simulink model "RemoteMicrogrid"  (R2025a)
settings: Solver=FixedStepAuto  StartTime=0.0  StopTime=8  FixedStep=Ts  MaxStep=1e-3  RelTol=1e-3
PreLoadFcn:
  | RemoteMicrogridInputData
undefined symbols (not defined in the file): BESS, ControlRoom, DiscIntNeverNeededParam, Grid, Load, Machine, Microgrid, MicrogridStatus, PV, relay1, T_on, Ts
libraries: ee_lib x53, fl_lib x39, eeGeneralControl x30, simulink x30, nesl_utility x26, nesl_utility_internal x19, slpidlib x7, eeTransforms x5, eeRmsMeasurement x4, eeTotalHarmonicDistorsion x4, batteryecm_lib x2, simulink_extras x2
(part 5 of 6)

== system RemoteMicrogrid/Diesel Substation, BESS, & Microgrid Controller/Microgrid Controller/Microgrid Supervisory Control/Transition and Dispatch Control/On.Unplanned_Islanding ==
  " Demux " : Demux  Outputs=1
  " Ground " : Ground
  " SFunction " : S-Function  Tag=Stateflow S-Function 9  FunctionName=sf_sfun  PortCounts=[1 6]  SFunctionDeploymentMode=off  EnableBusSupport=off
  " Terminator " : Terminator
  PCC : Outport
  loadDispatch : Outport  Port=2
  loadF2A : Outport  Port=3
  loadF2B : Outport  Port=4
  emergencyDispatch : Outport  Port=5
  wires:
  " SFunction "/2 -> PCC/1  "PCC"
  " SFunction "/3 -> loadDispatch/1  "loadDispatch"
  " SFunction "/4 -> loadF2A/1  "loadF2A"
  " SFunction "/5 -> loadF2B/1  "loadF2B"
  " SFunction "/6 -> emergencyDispatch/1  "emergencyDispatch"
  " Ground "/1 -> " SFunction "/1
  " Demux "/1 -> " Terminator "/1
  " SFunction "/1 -> " Demux "/1

== system RemoteMicrogrid/Operator Control Room/Microgrid Control/Protection & Power Tracking/Overcurrent relay ==
  Inport : Inport
  Data Type Conversion : DataTypeConversion  OutDataTypeStr=double  SaturateOnIntegerOverflow=off  RndMeth=Floor
  Delay : Delay  DelayLength=1
  Earth Protection Unit : Subsystem
  Enable : Gain  Gain=protectionEnable
  Fourier Analysis : Subsystem
  Mux1 : Mux  Inputs=2
  OR1 : Logic  Operator=OR  IconShape=distinctive  AllPortsSameDT=off  OutDataTypeStr=boolean
  Phase Protection Unit : Subsystem
  Trip Signal : Outport
  Relay Status : Outport  Port=2
  wires:
  Data Type Conversion/1 -> Enable/1
  Enable/1 -> Delay/1
  Delay/1 -> Trip Signal/1
  [Rer] -> Mux1/2
  [Rph] -> Mux1/1
  Mux1/1 -> Relay Status/1
  OR1/1 -> Data Type Conversion/1
  Inport/1 -> Fourier Analysis/1(Current)
  Fourier Analysis/1(Magnitude) -> [mag]
  Fourier Analysis/2(Angle) -> [iphi]
  [mag] -> Phase Protection Unit/1(Current)
  [mag] -> Earth Protection Unit/1(Mag)
  [iphi] -> Earth Protection Unit/2(Phi)
  Phase Protection Unit/1(Trip Signal) -> OR1/1, [Rph]
  Earth Protection Unit/1(Trip Signal) -> [Rer], OR1/2

== system RemoteMicrogrid/Operator Control Room/Performance and Power Quality/Load Performance /Subsystem4 ==
  Voltage : Inport
  Change Detector : eeGeneralControl/Change Detector  VariantControl=Variant1  LabelModeActiveChoice=Discrete  ChangeType=Rising edge  x0=0  Ts=Ts
  Change Detector1 : eeGeneralControl/Change Detector  VariantControl=Variant1  LabelModeActiveChoice=Discrete  ChangeType=Rising edge  x0=0  Ts=Ts
  Compare To Constant2 : simulink/Logic and Bit Operations/Compare To Constant  relop=<=  const=Microgrid.LoadVolatgeRMSLow  OutDataTypeStr=boolean
  Compare To Constant3 : simulink/Logic and Bit Operations/Compare To Constant  relop=>  const=Microgrid.LoadVolatgeRMSHigh  OutDataTypeStr=boolean
  VoltageLow : Outport
  VoltageHigh : Outport  Port=2
  wires:
  Change Detector/1 -> VoltageLow/1
  Compare To Constant2/1 -> Change Detector/1
  Voltage/1 -> Compare To Constant3/1, Compare To Constant2/1
  Change Detector1/1 -> VoltageHigh/1
  Compare To Constant3/1 -> Change Detector1/1

== system RemoteMicrogrid/Operator Control Room/Performance and Power Quality/Load Performance /start at 0.2 s2 ==
  In1 : Inport
  Constant : Constant
  Step : Step  Time=2.5  SampleTime=Ts
  Switch : Switch  Criteria=u2 > Threshold  Threshold=0.5  SaturateOnIntegerOverflow=off  InputSameDT=off
  u : Outport
  wires:
  In1/1 -> Switch/1
  Switch/1 -> u/1
  Constant/1 -> Switch/3
  Step/1 -> Switch/2

== system RemoteMicrogrid/Operator Control Room/Performance and Power Quality/Load Performance /start at 0.2 s4 ==
  In1 : Inport
  Constant : Constant  Value=0.491
  Step : Step  Time=2.5  SampleTime=Ts
  Switch : Switch  Criteria=u2 > Threshold  Threshold=0.5  SaturateOnIntegerOverflow=off  InputSameDT=off
  u : Outport
  wires:
  In1/1 -> Switch/1
  Switch/1 -> u/1
  Constant/1 -> Switch/3
  Step/1 -> Switch/2

== system RemoteMicrogrid/Operator Control Room/Performance and Power Quality/Load Performance /start at 0.2 s5 ==
  In1 : Inport
  Constant : Constant  Value=75
  Step : Step  Time=2.5  SampleTime=Ts
  Switch : Switch  Criteria=u2 > Threshold  Threshold=0.5  SaturateOnIntegerOverflow=off  InputSameDT=off
  u : Outport
  wires:
  Step/1 -> Switch/2
  Constant/1 -> Switch/3
  Switch/1 -> u/1
  In1/1 -> Switch/1

== system RemoteMicrogrid/Operator Control Room/Performance and Power Quality/Loss Calculation/start at 2.5 s ==
  ReactivePower : Inport
  Constant : Constant
  Step : Step  Time=2.5  SampleTime=Ts
  Switch : Switch  Criteria=u2 > Threshold  Threshold=0.5  SaturateOnIntegerOverflow=off  InputSameDT=off
  u : Outport
  wires:
  ReactivePower/1 -> Switch/1
  Switch/1 -> u/1
  Constant/1 -> Switch/3
  Step/1 -> Switch/2

== system RemoteMicrogrid/Operator Control Room/Performance and Power Quality/Loss Calculation/start at 2.5 s1 ==
  ActivePower : Inport
  Constant : Constant
  Step : Step  Time=2.5  SampleTime=Ts
  Switch : Switch  Criteria=u2 > Threshold  Threshold=0.5  SaturateOnIntegerOverflow=off  InputSameDT=off
  u : Outport
  wires:
  Step/1 -> Switch/2
  Constant/1 -> Switch/3
  Switch/1 -> u/1
  ActivePower/1 -> Switch/1

== system RemoteMicrogrid/Operator Control Room/Performance and Power Quality/Microgrid Power Quality /Subsystem ==
  Frequency : Inport
  Change Detector : eeGeneralControl/Change Detector  VariantControl=Variant1  LabelModeActiveChoice=Discrete  ChangeType=Rising edge  x0=0  Ts=Ts
  Change Detector1 : eeGeneralControl/Change Detector  VariantControl=Variant1  LabelModeActiveChoice=Discrete  ChangeType=Rising edge  x0=0  Ts=Ts
  Compare To Constant2 : simulink/Logic and Bit Operations/Compare To Constant  relop=<  const=Microgrid.FrequencyLow  OutDataTypeStr=boolean
  Compare To Constant3 : simulink/Logic and Bit Operations/Compare To Constant  relop=>  const=Microgrid.FrequencyHigh  OutDataTypeStr=boolean
  FrequencyLow : Outport
  FrequencyHigh : Outport  Port=2
  wires:
  Change Detector/1 -> FrequencyLow/1
  Compare To Constant2/1 -> Change Detector/1
  Frequency/1 -> Compare To Constant3/1, Compare To Constant2/1
  Change Detector1/1 -> FrequencyHigh/1
  Compare To Constant3/1 -> Change Detector1/1

== system RemoteMicrogrid/Operator Control Room/Performance and Power Quality/Microgrid Power Quality /Subsystem3 ==
  Voltage : Inport
  Change Detector : eeGeneralControl/Change Detector  VariantControl=Variant1  LabelModeActiveChoice=Discrete  ChangeType=Rising edge  x0=0  Ts=Ts
  Change Detector1 : eeGeneralControl/Change Detector  VariantControl=Variant1  LabelModeActiveChoice=Discrete  ChangeType=Rising edge  x0=0  Ts=Ts
  Compare To Constant2 : simulink/Logic and Bit Operations/Compare To Constant  relop=<=  const=Microgrid.VoltageLow  OutDataTypeStr=boolean
  Compare To Constant3 : simulink/Logic and Bit Operations/Compare To Constant  relop=>  const=Microgrid.VoltageHigh  OutDataTypeStr=boolean
  VoltageLow : Outport
  VoltageHigh : Outport  Port=2
  wires:
  Compare To Constant3/1 -> Change Detector/1
  Change Detector/1 -> VoltageHigh/1
  Voltage/1 -> Compare To Constant2/1, Compare To Constant3/1
  Compare To Constant2/1 -> Change Detector1/1
  Change Detector1/1 -> VoltageLow/1

== system RemoteMicrogrid/Operator Control Room/Performance and Power Quality/Microgrid Power Quality /start at 2 s ==
  In1 : Inport
  Constant : Constant  Value=60
  Step : Step  Time=2  SampleTime=Ts
  Switch : Switch  Criteria=u2 > Threshold  Threshold=0.5  SaturateOnIntegerOverflow=off  InputSameDT=off
  u : Outport
  wires:
  Step/1 -> Switch/2
  Constant/1 -> Switch/3
  Switch/1 -> u/1
  In1/1 -> Switch/1

== system RemoteMicrogrid/Operator Control Room/Performance and Power Quality/Microgrid Power Quality /start at 2 s1 ==
  In1 : Inport
  Constant : Constant
  Step : Step  Time=2  SampleTime=Ts
  Switch : Switch  Criteria=u2 > Threshold  Threshold=0.5  SaturateOnIntegerOverflow=off  InputSameDT=off
  u : Outport
  wires:
  Step/1 -> Switch/2
  Constant/1 -> Switch/3
  Switch/1 -> u/1
  In1/1 -> Switch/1

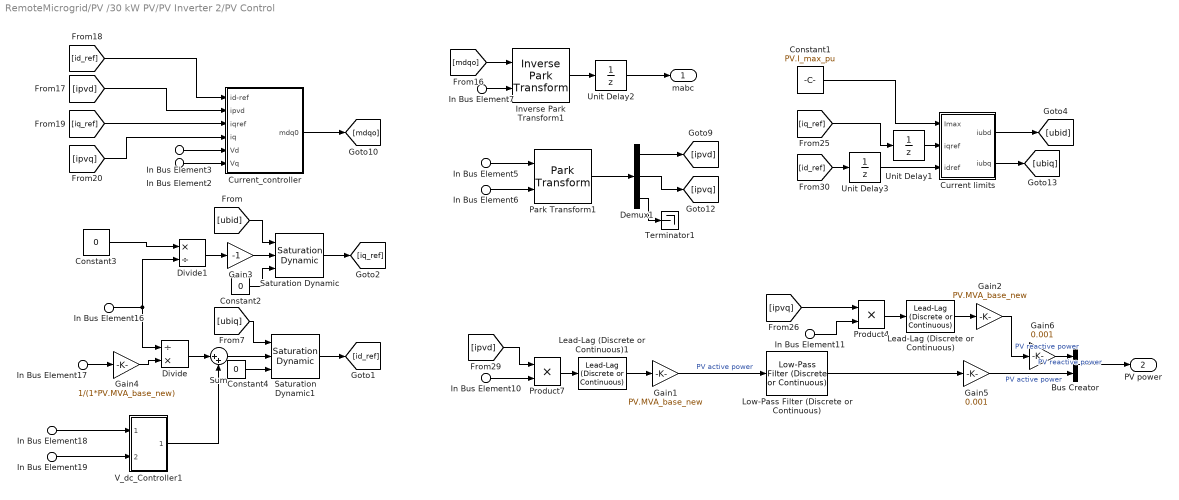
== system RemoteMicrogrid/PV /30 kW PV/PV Inverter 2/PV Control ==
  In Bus Element17 : Inport  PortName=PV_plant1  Element=Pref1
  In Bus Element18 : Inport  PortName=PV_plant1  Element=Vdc_measured
  In Bus Element19 : Inport  PortName=PV_plant1  Element=Vdc_ref
  In Bus Element{3,10..11,16} (4 alike) : Inport  Port=2  PortName=PV  Element=Vd
  In Bus Element2 : Inport  Port=2  PortName=PV  Element=Vq
  In Bus Element6 : Inport  Port=2  PortName=PV  Element=Theta
  In Bus Element7 : Inport  Port=2  PortName=PV  Element=Theta
  In Bus Element5 : Inport  Port=3  PortName=ipv1  Element=1
  Bus Creator : BusCreator  Inputs=2
  Constant1 : Constant  Value=PV.I_max_pu
  Constant2 : Constant  Value=0
  Constant3 : Constant  Value=0
  Constant4 : Constant  Value=0
  Current limits : Subsystem
  Current_controller : Subsystem
  Demux1 : Demux  Outputs=3
  Divide : Product  Inputs=/*
  Divide1 : Product  Inputs=*/
  Gain1 : Gain  Gain=PV.MVA_base_new
  Gain2 : Gain  Gain=PV.MVA_base_new
  Gain3 : Gain  Gain=-1
  Gain4 : Gain  Gain=1/(1*PV.MVA_base_new)
  Gain5 : Gain  Gain=0.001
  Gain6 : Gain  Gain=0.001
  Inverse Park Transform1 : eeTransforms/Inverse Park Transform  AxisAlignment=Q-axis  PowerInvariant=off
  Lead-Lag (Discrete or Continuous) : eeGeneralControl/Lead-Lag (Discrete or Continuous)  T1=0  T2=PV.t_sensor  B=inf  A=-inf  init_option=Inherited from block input  x0=0  Ts=Ts
      settings: LibrarySourceBlock=|
      | ee_sl_lib/General Control/Lead-Lag
      | (Discrete or Continuous)
  Lead-Lag (Discrete or Continuous)1 : eeGeneralControl/Lead-Lag (Discrete or Continuous)  T1=0  T2=PV.t_sensor  B=inf  A=-inf  init_option=Inherited from block input  x0=0  Ts=Ts
      settings: LibrarySourceBlock=|
      | ee_sl_lib/General Control/Lead-Lag
      | (Discrete or Continuous)
  Low-Pass Filter (Discrete or Continuous) : eeGeneralControl/Low-Pass Filter (Discrete or Continuous)  K=1  T=0.02  B=inf  A=-inf  init_option=Inherited from block input  x0=0  Ts=-1
  Park Transform1 : eeTransforms/Park Transform  AxisAlignment=Q-axis  PowerInvariant=off
  Product4 : Product
  Product7 : Product
  Saturation Dynamic : simulink/Discontinuities/Saturation Dynamic  OutMin=[]  OutMax=[]  OutDataTypeStr=Inherit: Same as second input  OutDataType=fixdt(1, 16)  OutScaling=2^-10  DoSatur=off
  Saturation Dynamic1 : simulink/Discontinuities/Saturation Dynamic  OutMin=[]  OutMax=[]  OutDataTypeStr=Inherit: Same as second input  OutDataType=fixdt(1, 16)  OutScaling=2^-10  DoSatur=off
  Sum : Sum  Inputs=|++
  Terminator1 : Terminator
  Unit Delay1 : UnitDelay  SampleTime=Ts  HasFrameUpgradeWarning=on
  Unit Delay2 : UnitDelay  SampleTime=Ts  HasFrameUpgradeWarning=on
  Unit Delay3 : UnitDelay  SampleTime=Ts  HasFrameUpgradeWarning=on
  V_dc_Controller1 : Subsystem
  mabc : Outport
  PV power : Outport  Port=2
  wires:
  [id_ref] -> Unit Delay3/1
  Current limits/2(iubq) -> [ubiq]
  Gain1/1 -> Low-Pass Filter (Discrete or Continuous)/1  "PV active power"
  Product4/1 -> Lead-Lag (Discrete or Continuous)/1
  Product7/1 -> Lead-Lag (Discrete or Continuous)1/1
  In Bus Element2/1 -> Current_controller/6(Vq)
  Current_controller/1(mdq0) -> [mdqo]
  Constant1/1 -> Current limits/1(Imax)
  Inverse Park Transform1/1 -> Unit Delay2/1
  Demux1/2 -> [ipvq]
  Unit Delay2/1 -> mabc/1
  Demux1/1 -> [ipvd]
  [ipvq] -> Product4/1
  Demux1/3 -> Terminator1/1
  [mdqo] -> Inverse Park Transform1/1
  Current limits/1(iubd) -> [ubid]
  Park Transform1/1 -> Demux1/1
  [id_ref] -> Current_controller/1(id-ref)
  [iq_ref] -> Unit Delay1/1
  In Bus Element3/1 -> Current_controller/5(Vd)
  Unit Delay1/1 -> Current limits/2(iqref)
  [iq_ref] -> Current_controller/3(iqref)
  [ipvq] -> Current_controller/4(iq)
  In Bus Element10/1 -> Product7/2
  In Bus Element6/1 -> Park Transform1/2
  In Bus Element7/1 -> Inverse Park Transform1/2
  [ipvd] -> Product7/1
  Unit Delay3/1 -> Current limits/3(idref)
  In Bus Element11/1 -> Product4/2
  [ipvd] -> Current_controller/2(ipvd)
  Lead-Lag (Discrete or Continuous)1/1 -> Gain1/1
  Lead-Lag (Discrete or Continuous)/1 -> Gain2/1
  Gain2/1 -> Gain6/1  "PV reactive power"
  In Bus Element5/1 -> Park Transform1/1
  Constant4/1 -> Saturation Dynamic1/3
  V_dc_Controller1/1(Out1) -> Sum/2
  Constant2/1 -> Saturation Dynamic/3
  [ubiq] -> Saturation Dynamic1/1
  In Bus Element19/1 -> V_dc_Controller1/2(In2)
  Gain3/1 -> Saturation Dynamic/2
  In Bus Element18/1 -> V_dc_Controller1/1(PV_plant1)
  Gain4/1 -> Divide/2
  Sum/1 -> Saturation Dynamic1/2
  [ubid] -> Saturation Dynamic/1
  Constant3/1 -> Divide1/1
  In Bus Element16/1 -> Divide1/2, Divide/1
  Saturation Dynamic1/1 -> [id_ref]
  Divide/1 -> Sum/1
  Divide1/1 -> Gain3/1
  Saturation Dynamic/1 -> [iq_ref]
  In Bus Element17/1 -> Gain4/1
  Bus Creator/1 -> PV power/1
  Gain5/1 -> Bus Creator/2  "PV active power"
  Gain6/1 -> Bus Creator/1  "PV reactive power"
  Low-Pass Filter (Discrete or Continuous)/1 -> Gain5/1

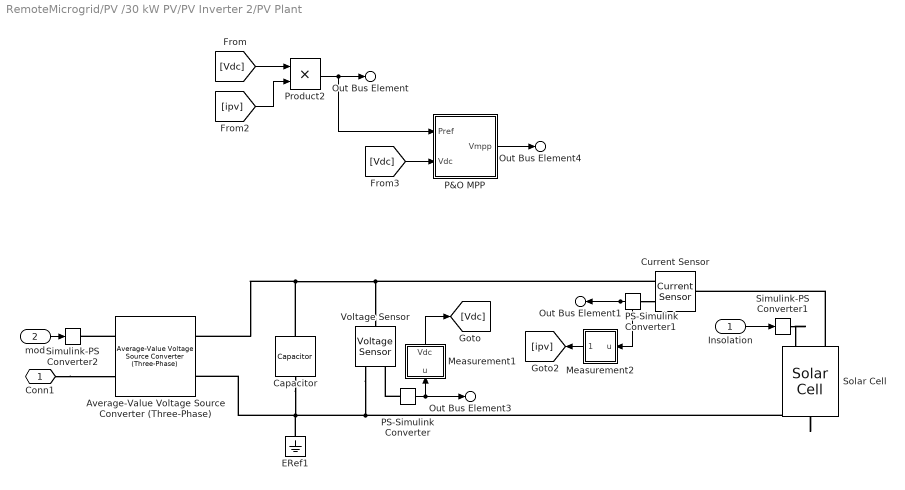
== system RemoteMicrogrid/PV /30 kW PV/PV Inverter 2/PV Plant ==
  Insolation : Inport
  mod : Inport  Port=2
  Average-Value Voltage Source Converter (Three-Phase) : ee_lib/Semiconductors & Converters/Converters/Average-Value Voltage Source Converter (Three-Phase)  port_option=ee.enum.threePhasePort.composite  frequency_option=ee.enum.converters.frequency.variable  input_option=ee.enum.converters.inputOption.ModWave  FRated=60 Hz  losses_parameterization=ee.enum.converters.losses.fixed  Pfixed=1 W  ks=0.01  kc1=1.7 V  kc2=0.01 Ohm  Ploss_vect=[100, 800, 1870, 3250, 4900] W  Irms_vect=[10, 100, 200, 300, 400] A  Vdc_nom=300 V  thermal_mass=30000 J/K  temperature_specify=off  temperature_priority=High  temperature=298.15 K  temperature_nominal_specify=off  temperature_nominal_value=1  temperature_nominal_unit=K
      settings: InternalSimscapePortConfiguration="{\"Bottom\":[],\"Left\":[{\"id\":\"ModWave\",\"label\":\"ModWave\",\"type\":\"input\"},{\"id\":\"N\",\"label\":\"~\",\"type\":\"foundation.electrical.three_phase\"}],\"Right\":[{\"id\":\"p\",\"label\":\"+\",\"type\":\"foundation.electrical.electrical\"},{\"id\":\"n\",\"label\":\"-\",\"type\":\"foundation.electrical.electrical\"}],\"Top\":[]}"
  Capacitor : fl_lib/Electrical/Electrical Elements/Capacitor  c=PV.C F  r=1e-6 Ohm  g=0 1/Ohm  i_specify=off  i_priority=None  i=0 A  i_nominal_specify=off  i_nominal_value=1  i_nominal_unit=A  v_specify=off  v_priority=None  v=6560*.5 V  v_nominal_specify=off  v_nominal_value=1  v_nominal_unit=V  vc_specify=on  vc_priority=None  vc=PV.Vdc V  vc_nominal_specify=off  vc_nominal_value=1  vc_nominal_unit=V
  Current Sensor : fl_lib/Electrical/Electrical Sensors/Current Sensor
  ERef1 : fl_lib/Electrical/Electrical Elements/Electrical Reference
  Measurement1 : Subsystem
  Measurement2 : Subsystem
  P&O MPP : Subsystem
  PS-Simulink Converter : nesl_utility/PS-Simulink Converter  PhysicalDomain=network_engine_domain  SubClassName=ps_output  LeftPortType=input  RightPortType=output  PseudoPeriodic=off  Frequencies=[]  VectorFormat=inherit  Unit=inherit  AffineConversion=off
  PS-Simulink Converter1 : nesl_utility/PS-Simulink Converter  PhysicalDomain=network_engine_domain  SubClassName=ps_output  LeftPortType=input  RightPortType=output  PseudoPeriodic=off  Frequencies=[]  VectorFormat=inherit  Unit=inherit  AffineConversion=off
  Product2 : Product
  Simulink-PS Converter1 : nesl_utility/Simulink-PS Converter  PhysicalDomain=network_engine_domain  SubClassName=ps_input  LeftPortType=input  RightPortType=output  PseudoPeriodic=off  Frequencies=[]  NoiseDistribution=none  NoiseParameters=[]  Unit=1  AffineConversion=off  FilteringAndDerivatives=provide  SimscapeFilterOrder=1  InputFilterTimeConstant=0.001  UdotUserProvided=0
  Simulink-PS Converter2 : nesl_utility/Simulink-PS Converter  PhysicalDomain=network_engine_domain  SubClassName=ps_input  LeftPortType=input  RightPortType=output  PseudoPeriodic=off  Frequencies=[]  NoiseDistribution=none  NoiseParameters=[]  Unit=1  AffineConversion=off  FilteringAndDerivatives=provide  SimscapeFilterOrder=1  InputFilterTimeConstant=0.001  UdotUserProvided=0
  Solar Cell : ee_lib/Sources/Solar Cell  prm=3  Isc=3.8 A  Voc=0.586 V  Is=Solar_cell.diode_saturation_current A  Is2=0 A  Iph=Solar_cell.solar_generated_current_AM A  Ir0=1000 W/m^2  ec=Solar_cell.quality_factor_i  N2=Solar_cell.quality_factor_j  Rs=Solar_cell.series_resistance Ohm  Rp=Solar_cell.parallel_resistance Ohm  N_series=PV.n_series_cell_panel*PV.n_series_panels_per_string  N_parallel=PV.n_parallel_strings_panel*PV.n_parallel_strings  TIPH1=Solar_cell.temp_cofficient 1/K  EG=Solar_cell.Eg eV  TXIS1=Solar_cell.temparature_exponent_Is1  TXIS2=Solar_cell.temparature_exponent_Is2  TRS1=Solar_cell.temparature_exponent_Rs  TRP1=Solar_cell.temparature_exponent_Rp  Tmeas=Solar_cell.measurement_temperature degC  TFIXED=Solar_cell.device_temperature degC  thermal_mass=100 J/K  initial_temperature=25 degC
  Voltage Sensor : fl_lib/Electrical/Electrical Sensors/Voltage Sensor
  Conn1 : PMIOPort  Side=Right
  Out Bus Element4 : Outport  PortName=PV_plant1  Element=Vdc_ref
  Out Bus Element : Outport  PortName=PV_plant1  Element=Pref1
  Out Bus Element3 : Outport  PortName=PV_plant1  Element=Vdc_measured
  Out Bus Element1 : Outport  PortName=PV_plant1  Element=ipv
  wires:
  PS-Simulink Converter1/1 -> Measurement2/1(u), Out Bus Element1/1
  Insolation/1 -> Simulink-PS Converter1/1
  [ipv] -> Product2/2
  PS-Simulink Converter/1 -> Measurement1/1(u), Out Bus Element3/1
  [Vdc] -> Product2/1
  mod/1 -> Simulink-PS Converter2/1
  Product2/1 -> P&O MPP/1(Pref), Out Bus Element/1
  P&O MPP/1(Vmpp) -> Out Bus Element4/1
  [Vdc] -> P&O MPP/2(Vdc)
  Measurement1/1(Vdc) -> [Vdc]
  Measurement2/1(Out1) -> [ipv]
  connections:
  PS-Simulink Converter/LConn1 -- Voltage Sensor/RConn1
  Capacitor/LConn1 -- Current Sensor/RConn2 -- Voltage Sensor/LConn1 -- Average-Value Voltage Source Converter (Three-Phase)/RConn1
  Voltage Sensor/RConn2 -- ERef1/LConn1 -- Capacitor/RConn1 -- Average-Value Voltage Source Converter (Three-Phase)/RConn2 -- Solar Cell/RConn1
  Average-Value Voltage Source Converter (Three-Phase)/LConn1 -- Simulink-PS Converter2/RConn1
  Solar Cell/LConn2 -- Current Sensor/LConn1
  Conn1/RConn1 -- Average-Value Voltage Source Converter (Three-Phase)/LConn2
  PS-Simulink Converter1/LConn1 -- Current Sensor/RConn1
  Simulink-PS Converter1/RConn1 -- Solar Cell/LConn1

== system RemoteMicrogrid/Operator Control Room/Microgrid Control/Protection & Power Tracking/Overcurrent relay/Earth Protection Unit ==
  Mag : Inport
  Phi : Inport  Port=2
  Compare To Constant1 : simulink/Logic and Bit Operations/Compare To Constant  relop=>=  const=1  OutDataTypeStr=boolean
  Constant10 : Constant  Value=0  OutDataTypeStr=boolean
  Constant7 : Constant  Value=0  OutDataTypeStr=double
  Data Type Conversion1 : DataTypeConversion  OutDataTypeStr=double  SaturateOnIntegerOverflow=off  RndMeth=Floor
  Delay1 : Delay  DelayLength=1
  Gain1 : Gain  Gain=1/(ethPickUp)
  GreaterThan2 : RelationalOperator  Operator=<=  OutDataTypeStr=boolean  RndMeth=Simplest  InputSameDT=off
  Integrator (Discrete or Continuous)1 : eeGeneralControl/Integrator (Discrete or Continuous)  LabelModeActiveChoice=Discrete  ExternalReset=falling  LimitType=Anti-windup  B=inf  A=-inf  Ts=sampleTime
  Operating Time : Subsystem
  S-R Flip-Flop2 : simulink_extras/Flip Flops/S-R Flip-Flop  initial_condition=0
  Scope : Scope
      settings: ActiveDisplayYMinimum=-2E-12  ActiveDisplayYMaximum=1.4E-11  DataLoggingVariableName=ScopeData3
  Terminator3 : Terminator
  Zero Sequence Current : Subsystem
  Trip Signal : Outport
  wires:
  Gain1/1 -> Operating Time/2(Plug Setting), Compare To Constant1/1
  Compare To Constant1/1 -> Data Type Conversion1/1
  GreaterThan2/1 -> Delay1/1, S-R Flip-Flop2/1
  Delay1/1 -> Integrator (Discrete or Continuous)1/2
  Constant10/1 -> S-R Flip-Flop2/2
  Zero Sequence Current/1(I0) -> Scope/1, Gain1/1, Operating Time/1(Zero Sequence Current)
  Data Type Conversion1/1 -> Integrator (Discrete or Continuous)1/1
  Integrator (Discrete or Continuous)1/1 -> GreaterThan2/2
  Operating Time/1(Operating Time) -> GreaterThan2/1
  S-R Flip-Flop2/2 -> Terminator3/1
  Constant7/1 -> Integrator (Discrete or Continuous)1/3
  Phi/1 -> Zero Sequence Current/2(Phi)
  Mag/1 -> Zero Sequence Current/1(Mag)
  S-R Flip-Flop2/1 -> Trip Signal/1

== system RemoteMicrogrid/Operator Control Room/Microgrid Control/Protection & Power Tracking/Overcurrent relay/Fourier Analysis ==
  Current : Inport
  Add1 : Sum  Inputs=-+
  Delay3 : Delay  DelayLength=1
  Fourier Analysis2 : eeGeneralControl/Fourier Analysis  f=ratedFrequency  n=[1]  M0=0  Ph0=0  BufferSize=8192  Ts=sampleTime
  Gain : Gain  Gain=1/sqrt(2)
  Moving Average : eeGeneralControl/Moving Average  VariantControl=Variant1  LabelModeActiveChoice=Discrete  f=50  x0=0  BufferSize=8192  Ts=sampleTime
  Scope : Scope
      settings: ActiveDisplayYMinimum=-0.51657  ActiveDisplayYMaximum=5.15314  DataLoggingVariableName=ScopeData2
  Magnitude : Outport
  Angle : Outport  Port=2
  wires:
  Delay3/1 -> Add1/2, Moving Average/1
  Current/1 -> Delay3/1
  Fourier Analysis2/2 -> Angle/1
  Moving Average/1 -> Add1/1
  Add1/1 -> Fourier Analysis2/1
  Fourier Analysis2/1 -> Gain/1
  Gain/1 -> Scope/1, Magnitude/1

== system RemoteMicrogrid/Operator Control Room/Microgrid Control/Protection & Power Tracking/Overcurrent relay/Phase Protection Unit ==
  Current : Inport
  Compare To Constant : simulink/Logic and Bit Operations/Compare To Constant  relop=>=  const=1  OutDataTypeStr=boolean
  Constant2 : Constant  Value=0  OutDataTypeStr=boolean
  Constant4 : Constant  Value=0  OutDataTypeStr=boolean
  Constant8 : Constant  Value=0  OutDataTypeStr=double
  Data Type Conversion2 : DataTypeConversion  OutDataTypeStr=double  SaturateOnIntegerOverflow=off  RndMeth=Floor
  Delay2 : Delay  DelayLength=1
  Demux : Demux  Outputs=3
  Gain2 : Gain  Gain=1/(phPickUp)
  GreaterThan : RelationalOperator  Operator=<=  OutDataTypeStr=boolean  RndMeth=Simplest  InputSameDT=off
  Integrator (Discrete or Continuous) : eeGeneralControl/Integrator (Discrete or Continuous)  LabelModeActiveChoice=Discrete  ExternalReset=falling  LimitType=Anti-windup  B=inf  A=-inf  Ts=sampleTime
  OR : Logic  Operator=OR  Inputs=3  IconShape=distinctive  AllPortsSameDT=off  OutDataTypeStr=boolean
  "Operating time " : Subsystem
  S-R Flip-Flop : simulink_extras/Flip Flops/S-R Flip-Flop  initial_condition=0
  Switch1 : Switch  Criteria=u2 > Threshold  OutDataTypeStr=boolean  SaturateOnIntegerOverflow=off  InputSameDT=off
  Terminator2 : Terminator
  Trip Signal : Outport
  wires:
  Data Type Conversion2/1 -> Integrator (Discrete or Continuous)/1, Switch1/2
  Gain2/1 -> "Operating time "/2(plugSetting), Compare To Constant/1
  Constant2/1 -> Switch1/3
  Demux/2 -> OR/2
  OR/1 -> Data Type Conversion2/1
  Integrator (Discrete or Continuous)/1 -> GreaterThan/2
  Demux/3 -> OR/3
  Current/1 -> Gain2/1, "Operating time "/1(Current)
  GreaterThan/1 -> Switch1/1
  "Operating time "/1(Operating Time) -> GreaterThan/1
  Constant4/1 -> S-R Flip-Flop/2
  S-R Flip-Flop/2 -> Terminator2/1
  Switch1/1 -> S-R Flip-Flop/1
  Demux/1 -> OR/1
  Constant8/1 -> Integrator (Discrete or Continuous)/3
  Compare To Constant/1 -> Demux/1
  S-R Flip-Flop/1 -> Trip Signal/1, [Rph]
  Delay2/1 -> Integrator (Discrete or Continuous)/2
  [Rph] -> Delay2/1

== system RemoteMicrogrid/PV /30 kW PV/PV Inverter 2/PV Control/Current limits ==
  Imax : Inport
  iqref : Inport  Port=2
  idref : Inport  Port=3
  Constant8 : Constant  Value=0
  Constant9 : Constant  Value=0
  Sqrt : Sqrt
  Sqrt1 : Sqrt
  Square{1..4} (4 alike) : Math  Operator=square
  Step2 : Step  Time=T_on  SampleTime=Ts
  Step3 : Step  Time=T_on  SampleTime=Ts
  Sum6 : Sum  Inputs=|+-
  Sum9 : Sum  Inputs=|+-
  Switch1 : Switch  Threshold=.01  SaturateOnIntegerOverflow=off  InputSameDT=off
  Switch2 : Switch  Threshold=.01  SaturateOnIntegerOverflow=off  InputSameDT=off
  iubd : Outport
  iubq : Outport  Port=2
  wires:
  Sum9/1 -> Switch2/1
  Step3/1 -> Switch2/2
  Step2/1 -> Switch1/2
  Switch2/1 -> Sqrt1/1
  Square1/1 -> Sum6/1
  Switch1/1 -> Sqrt/1
  iqref/1 -> Square2/1
  Square3/1 -> Sum9/1
  Sum6/1 -> Switch1/1
  Square2/1 -> Sum6/2
  Constant8/1 -> Switch1/3
  Square4/1 -> Sum9/2
  Constant9/1 -> Switch2/3
  Sqrt/1 -> iubd/1
  Imax/1 -> Square3/1, Square1/1
  Sqrt1/1 -> iubq/1
  idref/1 -> Square4/1

== system RemoteMicrogrid/PV /30 kW PV/PV Inverter 2/PV Control/Current_controller ==
  id-ref : Inport
  ipvd : Inport  Port=2
  iqref : Inport  Port=3
  iq : Inport  Port=4
  Vd : Inport  Port=5
  Vq : Inport  Port=6
  Constant4 : Constant  Value=0
  Gain1 : Gain  Gain=2*1*pi*60*PV.L/PV.z_base
  Gain2 : Gain  Gain=2*1*pi*60*PV.L/PV.z_base
  Mux1 : Mux  Inputs=3
  PID Controller : slpidlib/PID Controller  Controller=PID  Form=Parallel  TimeDomain=Discrete-time  UseExternalTs=off  SampleTime=-1  IntegratorMethod=Forward Euler  FilterMethod=Forward Euler  ControllerParametersSource=internal  P=PV.Kp_ic  I=PV.Ki_ic  UseKiTs=off  D=PV.Kd  UseExternalDerivativeSource=off  N=100  UseFilter=on  TunerSelectOption=Transfer Function Based (PID Tuner App)  InitialConditionSource=internal  InitialConditionForIntegrator=0.9  InitialConditionForFilter=0  DifferentiatorICPrevScaledInput=0  ExternalReset=none  TrackingMode=off  Kt=1  LimitOutput=off  SatLimitsSource=internal  UpperSaturationLimit=inf  LowerSaturationLimit=-inf  LinearizeAsGain=on  AntiWindupMode=none  Kb=1  LimitIntegrator=off  UpperIntegratorSaturationLimit=inf  LowerIntegratorSaturationLimit=-inf  POutMin=[]  POutMax=[]  IOutMin=[]  IOutMax=[]  DOutMin=[]  DOutMax=[]  NOutMin=[]  NOutMax=[]  SumOutMin=[]  SumOutMax=[]  SaturationOutMin=[]  SaturationOutMax=[]  PParamMin=[]  PParamMax=[]  IParamMin=[]  IParamMax=[]  DParamMin=[]  DParamMax=[]  NParamMin=[]  NParamMax=[]  KbParamMin=[]  KbParamMax=[]  KtParamMin=[]  KtParamMax=[]  KbOutMin=[]  KbOutMax=[]  KtOutMin=[]  KtOutMax=[]  IntegratorOutMin=[]  IntegratorOutMax=[]  FilterOutMin=[]  FilterOutMax=[]  SumI1OutMin=[]  SumI1OutMax=[]  SumI2OutMin=[]  SumI2OutMax=[]  SumI3OutMin=[]  SumI3OutMax=[]  SumI4OutMin=[]  SumI4OutMax=[]  SumDOutMin=[]  SumDOutMax=[]  DifferentiatorOutMin=[]  DifferentiatorOutMax=[]  FilterDiffOutCoefMin=[]  FilterDiffOutCoefMax=[]  ReciprocalOutMin=[]  ReciprocalOutMax=[]  SumDenOutMin=[]  SumDenOutMax=[]  SumNumOutMin=[]  SumNumOutMax=[]  DivideOutMin=[]  DivideOutMax=[]  UdiffTsProdOutMin=[]  UdiffTsProdOutMax=[]  NTsProdOutMin=[]  NTsProdOutMax=[]  UintegralTsProdOutMin=[]  UintegralTsProdOutMax=[]  UngainTsProdOutMin=[]  UngainTsProdOutMax=[]  ClampingZeroOutDataTypeStr=Inherit: Inherit via back propagation  ClampingZeroOutMin=[]  ClampingZeroOutMax=[]  FilterDenConstantOutDataTypeStr=Inherit: Inherit via back propagation  FilterDenConstantOutMin=[]  FilterDenConstantOutMax=[]  PCopyOutDataTypeStr=Inherit: Inherit via back propagation  PCopyOutMin=[]  PCopyOutMax=[]  NCopyOutDataTypeStr=Inherit: Inherit via back propagation  NCopyOutMin=[]  NCopyOutMax=[]  IntegratorContinuousStateAttributes=''  IntegratorStateMustResolveToSignalObject=off  IntegratorRTWStateStorageClass=Auto  FilterContinuousStateAttributes=''  FilterStateMustResolveToSignalObject=off  FilterRTWStateStorageClass=Auto  ParallelPVariant=InternalParameters  IdealPVariant=Disabled  IVariant=InternalParameters  DVariant=InternalParameters  IntegratorVariant=Discrete  SatVariant=Disabled  AWVariant=Passthrough  PCopyVariant=Disabled  TRVariant=Disabled  FdbkBlocksVariant=Forward  IdealPFdbkVariant=Disabled  SatFdbkVariant=Disabled  DerivativeFilterVariant=ForwardEulerFilter  NVariant=InternalParameters  NCopyVariant=Disabled  FilterICVariant=InternalICsFilter  IntegratorICVariant=InternalICs  ExternalResetVariant=Disabled  TRSumVariant=Passthrough  SumFdbkVariant=Disabled  SumVariant=Sum_PID  TsampFilterVariant=InternalTs  TsampNgainVariant=Passthrough  TsampIntegralVariant=Disabled_SignalSpec  ExternalSaturationOutDataTypeStr=Inherit: Same as second input  DerivativeSourceVariant=ErrorSignal  PreIntVariant=InternalPreInt
  PID Controller1 : slpidlib/PID Controller  Controller=PID  Form=Parallel  TimeDomain=Discrete-time  UseExternalTs=off  SampleTime=-1  IntegratorMethod=Forward Euler  FilterMethod=Forward Euler  ControllerParametersSource=internal  P=PV.Kp_ic  I=PV.Ki_ic  UseKiTs=off  D=PV.Kd  UseExternalDerivativeSource=off  N=100  UseFilter=on  TunerSelectOption=Transfer Function Based (PID Tuner App)  InitialConditionSource=internal  InitialConditionForIntegrator=1.05  InitialConditionForFilter=0  DifferentiatorICPrevScaledInput=0  ExternalReset=none  TrackingMode=off  Kt=1  LimitOutput=off  SatLimitsSource=internal  UpperSaturationLimit=inf  LowerSaturationLimit=-inf  LinearizeAsGain=on  AntiWindupMode=none  Kb=1  LimitIntegrator=off  UpperIntegratorSaturationLimit=inf  LowerIntegratorSaturationLimit=-inf  POutMin=[]  POutMax=[]  IOutMin=[]  IOutMax=[]  DOutMin=[]  DOutMax=[]  NOutMin=[]  NOutMax=[]  SumOutMin=[]  SumOutMax=[]  SaturationOutMin=[]  SaturationOutMax=[]  PParamMin=[]  PParamMax=[]  IParamMin=[]  IParamMax=[]  DParamMin=[]  DParamMax=[]  NParamMin=[]  NParamMax=[]  KbParamMin=[]  KbParamMax=[]  KtParamMin=[]  KtParamMax=[]  KbOutMin=[]  KbOutMax=[]  KtOutMin=[]  KtOutMax=[]  IntegratorOutMin=[]  IntegratorOutMax=[]  FilterOutMin=[]  FilterOutMax=[]  SumI1OutMin=[]  SumI1OutMax=[]  SumI2OutMin=[]  SumI2OutMax=[]  SumI3OutMin=[]  SumI3OutMax=[]  SumI4OutMin=[]  SumI4OutMax=[]  SumDOutMin=[]  SumDOutMax=[]  DifferentiatorOutMin=[]  DifferentiatorOutMax=[]  FilterDiffOutCoefMin=[]  FilterDiffOutCoefMax=[]  ReciprocalOutMin=[]  ReciprocalOutMax=[]  SumDenOutMin=[]  SumDenOutMax=[]  SumNumOutMin=[]  SumNumOutMax=[]  DivideOutMin=[]  DivideOutMax=[]  UdiffTsProdOutMin=[]  UdiffTsProdOutMax=[]  NTsProdOutMin=[]  NTsProdOutMax=[]  UintegralTsProdOutMin=[]  UintegralTsProdOutMax=[]  UngainTsProdOutMin=[]  UngainTsProdOutMax=[]  ClampingZeroOutDataTypeStr=Inherit: Inherit via back propagation  ClampingZeroOutMin=[]  ClampingZeroOutMax=[]  FilterDenConstantOutDataTypeStr=Inherit: Inherit via back propagation  FilterDenConstantOutMin=[]  FilterDenConstantOutMax=[]  PCopyOutDataTypeStr=Inherit: Inherit via back propagation  PCopyOutMin=[]  PCopyOutMax=[]  NCopyOutDataTypeStr=Inherit: Inherit via back propagation  NCopyOutMin=[]  NCopyOutMax=[]  IntegratorContinuousStateAttributes=''  IntegratorStateMustResolveToSignalObject=off  IntegratorRTWStateStorageClass=Auto  FilterContinuousStateAttributes=''  FilterStateMustResolveToSignalObject=off  FilterRTWStateStorageClass=Auto  ParallelPVariant=InternalParameters  IdealPVariant=Disabled  IVariant=InternalParameters  DVariant=InternalParameters  IntegratorVariant=Discrete  SatVariant=Disabled  AWVariant=Passthrough  PCopyVariant=Disabled  TRVariant=Disabled  FdbkBlocksVariant=Forward  IdealPFdbkVariant=Disabled  SatFdbkVariant=Disabled  DerivativeFilterVariant=ForwardEulerFilter  NVariant=InternalParameters  NCopyVariant=Disabled  FilterICVariant=InternalICsFilter  IntegratorICVariant=InternalICs  ExternalResetVariant=Disabled  TRSumVariant=Passthrough  SumFdbkVariant=Disabled  SumVariant=Sum_PID  TsampFilterVariant=InternalTs  TsampNgainVariant=Passthrough  TsampIntegralVariant=Disabled_SignalSpec  ExternalSaturationOutDataTypeStr=Inherit: Same as second input  DerivativeSourceVariant=ErrorSignal  PreIntVariant=InternalPreInt
  Sum1 : Sum  Inputs=|+-
  Sum3 : Sum  Inputs=|++-
  Sum4 : Sum  Inputs=|+++
  Sum5 : Sum  Inputs=|+-
  mdq0 : Outport
  wires:
  PID Controller/1 -> Sum3/2
  Sum3/1 -> Mux1/1
  Gain2/1 -> Sum3/3
  ipvd/1 -> Gain1/1, Sum1/2
  id-ref/1 -> Sum1/1
  Gain1/1 -> Sum4/3
  Vq/1 -> Sum4/2
  iq/1 -> Gain2/1, Sum5/2
  Sum1/1 -> PID Controller/1
  Vd/1 -> Sum3/1
  Constant4/1 -> Mux1/3
  Sum5/1 -> PID Controller1/1
  iqref/1 -> Sum5/1
  PID Controller1/1 -> Sum4/1
  Sum4/1 -> Mux1/2
  Mux1/1 -> mdq0/1

== system RemoteMicrogrid/PV /30 kW PV/PV Inverter 2/PV Control/V_dc_Controller1 ==
  PV_plant1 : Inport
  In2 : Inport  Port=2
  Gain : Gain  Gain=1/PV.Vdc_base
  PID Controller : slpidlib/PID Controller  Controller=PID  Form=Parallel  TimeDomain=Discrete-time  UseExternalTs=off  SampleTime=-1  IntegratorMethod=Forward Euler  FilterMethod=Forward Euler  ControllerParametersSource=internal  P=PV.Kp_v  I=PV.Ki_v  UseKiTs=off  D=PV.Kd_v  UseExternalDerivativeSource=off  N=100  UseFilter=on  TunerSelectOption=Transfer Function Based (PID Tuner App)  ZeroCross=off  InitialConditionSource=internal  InitialConditionForIntegrator=0  InitialConditionForFilter=0  DifferentiatorICPrevScaledInput=0  ExternalReset=none  TrackingMode=off  Kt=1  LimitOutput=off  SatLimitsSource=internal  UpperSaturationLimit=inf  LowerSaturationLimit=-inf  LinearizeAsGain=on  AntiWindupMode=none  Kb=1  LimitIntegrator=off  UpperIntegratorSaturationLimit=inf  LowerIntegratorSaturationLimit=-inf  POutMin=[]  POutMax=[]  IOutMin=[]  IOutMax=[]  DOutMin=[]  DOutMax=[]  NOutMin=[]  NOutMax=[]  SumOutMin=[]  SumOutMax=[]  SaturationOutMin=[]  SaturationOutMax=[]  PParamMin=[]  PParamMax=[]  IParamMin=[]  IParamMax=[]  DParamMin=[]  DParamMax=[]  NParamMin=[]  NParamMax=[]  KbParamMin=[]  KbParamMax=[]  KtParamMin=[]  KtParamMax=[]  KbOutMin=[]  KbOutMax=[]  KtOutMin=[]  KtOutMax=[]  IntegratorOutMin=[]  IntegratorOutMax=[]  FilterOutMin=[]  FilterOutMax=[]  SumI1OutMin=[]  SumI1OutMax=[]  SumI2OutMin=[]  SumI2OutMax=[]  SumI3OutMin=[]  SumI3OutMax=[]  SumI4OutMin=[]  SumI4OutMax=[]  SumDOutMin=[]  SumDOutMax=[]  DifferentiatorOutMin=[]  DifferentiatorOutMax=[]  FilterDiffOutCoefMin=[]  FilterDiffOutCoefMax=[]  ReciprocalOutMin=[]  ReciprocalOutMax=[]  SumDenOutMin=[]  SumDenOutMax=[]  SumNumOutMin=[]  SumNumOutMax=[]  DivideOutMin=[]  DivideOutMax=[]  UdiffTsProdOutMin=[]  UdiffTsProdOutMax=[]  NTsProdOutMin=[]  NTsProdOutMax=[]  UintegralTsProdOutMin=[]  UintegralTsProdOutMax=[]  UngainTsProdOutMin=[]  UngainTsProdOutMax=[]  ClampingZeroOutDataTypeStr=Inherit: Inherit via back propagation  ClampingZeroOutMin=[]  ClampingZeroOutMax=[]  FilterDenConstantOutDataTypeStr=Inherit: Inherit via back propagation  FilterDenConstantOutMin=[]  FilterDenConstantOutMax=[]  PCopyOutDataTypeStr=Inherit: Inherit via back propagation  PCopyOutMin=[]  PCopyOutMax=[]  NCopyOutDataTypeStr=Inherit: Inherit via back propagation  NCopyOutMin=[]  NCopyOutMax=[]  IntegratorContinuousStateAttributes=''  IntegratorStateMustResolveToSignalObject=off  IntegratorRTWStateStorageClass=Auto  FilterContinuousStateAttributes=''  FilterStateMustResolveToSignalObject=off  FilterRTWStateStorageClass=Auto  ParallelPVariant=InternalParameters  IdealPVariant=Disabled  IVariant=InternalParameters  DVariant=InternalParameters  IntegratorVariant=Discrete  SatVariant=Disabled  AWVariant=Passthrough  PCopyVariant=Disabled  TRVariant=Disabled  FdbkBlocksVariant=Forward  IdealPFdbkVariant=Disabled  SatFdbkVariant=Disabled  DerivativeFilterVariant=ForwardEulerFilter  NVariant=InternalParameters  NCopyVariant=Disabled  FilterICVariant=InternalICsFilter  IntegratorICVariant=InternalICs  ExternalResetVariant=Disabled  TRSumVariant=Passthrough  SumFdbkVariant=Disabled  SumVariant=Sum_PID  TsampFilterVariant=InternalTs  TsampNgainVariant=Passthrough  TsampIntegralVariant=Disabled_SignalSpec  ExternalSaturationOutDataTypeStr=Inherit: Same as second input  DerivativeSourceVariant=ErrorSignal  PreIntVariant=InternalPreInt
  Sum : Sum  Inputs=|+-
  Out1 : Outport
  wires:
  PV_plant1/1 -> Sum/1
  In2/1 -> Sum/2
  PID Controller/1 -> Out1/1
  Gain/1 -> PID Controller/1
  Sum/1 -> Gain/1

== system RemoteMicrogrid/PV /30 kW PV/PV Inverter 2/PV Plant/Measurement1 ==
  u : Inport
  Lead-Lag (Discrete or Continuous) : eeGeneralControl/Lead-Lag (Discrete or Continuous)  T1=0  T2=PV.t_sensor  B=inf  A=-inf  init_option=Inherited from block input  x0=0  Ts=Ts
      settings: LibrarySourceBlock=|
      | ee_sl_lib/General Control/Lead-Lag
      | (Discrete or Continuous)
  Vdc : Outport
  wires:
  Lead-Lag (Discrete or Continuous)/1 -> Vdc/1
  u/1 -> Lead-Lag (Discrete or Continuous)/1

== system RemoteMicrogrid/PV /30 kW PV/PV Inverter 2/PV Plant/Measurement2 ==
  u : Inport
  Lead-Lag (Discrete or Continuous) : eeGeneralControl/Lead-Lag (Discrete or Continuous)  T1=0  T2=PV.t_sensor  B=inf  A=-inf  init_option=Inherited from block input  x0=0  Ts=Ts
      settings: LibrarySourceBlock=|
      | ee_sl_lib/General Control/Lead-Lag
      | (Discrete or Continuous)
  Out1 : Outport
  wires:
  Lead-Lag (Discrete or Continuous)/1 -> Out1/1
  u/1 -> Lead-Lag (Discrete or Continuous)/1

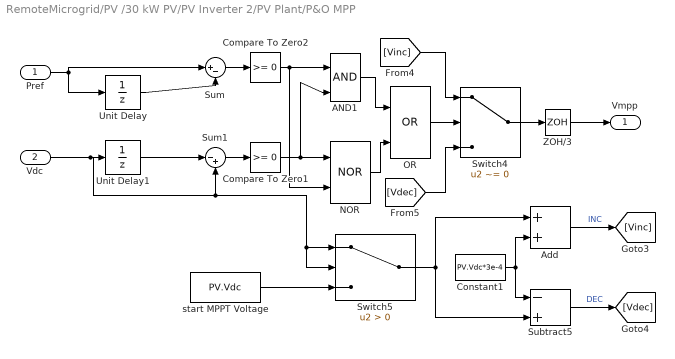
== system RemoteMicrogrid/PV /30 kW PV/PV Inverter 2/PV Plant/P&O MPP ==
  Pref : Inport
  Vdc : Inport  Port=2
  AND1 : Logic  IconShape=distinctive  AllPortsSameDT=off  OutDataTypeStr=boolean
  Add : Sum
  Compare To Zero1 : simulink/Logic and Bit Operations/Compare To Zero  relop=>=  OutDataTypeStr=boolean
  Compare To Zero2 : simulink/Logic and Bit Operations/Compare To Zero  relop=>=  OutDataTypeStr=boolean
  Constant1 : Constant  Value=PV.Vdc*3e-4
  NOR : Logic  Operator=NOR  IconShape=distinctive  AllPortsSameDT=off  OutDataTypeStr=boolean
  OR : Logic  Operator=OR  IconShape=distinctive  AllPortsSameDT=off  OutDataTypeStr=boolean
  Subtract5 : Sum  Inputs=-+
  Sum : Sum  Inputs=|+-
  Sum1 : Sum  Inputs=|-+
  Switch4 : Switch  Criteria=u2 ~= 0  SaturateOnIntegerOverflow=off  InputSameDT=off
  Switch5 : Switch  Criteria=u2 > Threshold  SaturateOnIntegerOverflow=off  InputSameDT=off
  Unit Delay : UnitDelay  InitialCondition=PV.Vdc  SampleTime=10*Ts  HasFrameUpgradeWarning=on
  Unit Delay1 : UnitDelay  InitialCondition=PV.Vdc  SampleTime=10*Ts  HasFrameUpgradeWarning=on
  ZOH/3 : ZeroOrderHold  SampleTime=100*Ts
  start MPPT Voltage : Constant  Value=PV.Vdc  SampleTime=Ts
  Vmpp : Outport  VectorParamsAs1DForOutWhenUnconnected=off
  wires:
  OR/1 -> Switch4/2
  Compare To Zero1/1 -> NOR/1, AND1/2
  start MPPT Voltage/1 -> Switch5/3
  Compare To Zero2/1 -> NOR/2, AND1/1
  Pref/1 -> Unit Delay/1, Sum/1
  Switch5/1 -> Add/1, Subtract5/2
  Constant1/1 -> Add/2, Subtract5/1
  Vdc/1 -> Switch5/2, Switch5/1, Sum1/2, Unit Delay1/1
  Unit Delay1/1 -> Sum1/1
  Add/1 -> [Vinc]  "INC"
  NOR/1 -> OR/2
  Subtract5/1 -> [Vdec]  "DEC"
  [Vdec] -> Switch4/3
  Switch4/1 -> ZOH/3/1
  Sum1/1 -> Compare To Zero1/1
  Sum/1 -> Compare To Zero2/1
  AND1/1 -> OR/1
  Unit Delay/1 -> Sum/2
  ZOH/3/1 -> Vmpp/1
  [Vinc] -> Switch4/1

== system RemoteMicrogrid/Operator Control Room/Microgrid Control/Protection & Power Tracking/Overcurrent relay/Earth Protection Unit/Operating Time ==
  Zero Sequence Current : Inport
  Plug Setting : Inport  Port=2
  Constant1 : Constant  Value=ethTimeSetting
  Constant11 : Constant  Value=relayCharacteristicEarth
  Constant6 : Constant  Value=relayCharacteristicEarth
  Lookup table : Subsystem
  Standard Characteristics : MATLAB Function  TreatAsAtomicUnit=on
  Switch2 : Switch  Threshold=7  SaturateOnIntegerOverflow=off  InputSameDT=off
  Operating Time : Outport
  wires:
  Constant1/1 -> Standard Characteristics/2(timeSetting)
  Lookup table/1(Oeprating Time) -> Switch2/1
  Constant6/1 -> Standard Characteristics/3(relayCharacteristic)
  Plug Setting/1 -> Standard Characteristics/1(plugSetting)
  Standard Characteristics/1(operatingTime) -> Switch2/3
  Constant11/1 -> Switch2/2
  Switch2/1 -> Operating Time/1
  Zero Sequence Current/1 -> Lookup table/1(Current)

== system RemoteMicrogrid/Operator Control Room/Microgrid Control/Protection & Power Tracking/Overcurrent relay/Earth Protection Unit/Zero Sequence Current ==
  Mag : Inport
  Phi : Inport  Port=2
  Add : Sum  Inputs=+++
  Complex to Magnitude-Angle : ComplexToMagnitudeAngle  Output=Magnitude
  Demux1 : Demux  Outputs=3
  Gain : Gain  Gain=1/3
  Magnitude-Angle to Complex : MagnitudeAngleToComplex
  I0 : Outport
  wires:
  Demux1/2 -> Add/2
  Demux1/3 -> Add/3
  Phi/1 -> Magnitude-Angle to Complex/2
  Complex to Magnitude-Angle/1 -> Gain/1
  Demux1/1 -> Add/1
  Mag/1 -> Magnitude-Angle to Complex/1
  Magnitude-Angle to Complex/1 -> Demux1/1
  Add/1 -> Complex to Magnitude-Angle/1
  Gain/1 -> I0/1

== system RemoteMicrogrid/Operator Control Room/Microgrid Control/Protection & Power Tracking/Overcurrent relay/Phase Protection Unit/Operating time  ==
  Current : Inport
  plugSetting : Inport  Port=2
  Constant : Constant  Value=phTimeSetting  VectorParams1D=off
  Constant3 : Constant  Value=relayCharacteristicPhase
  Constant9 : Constant  Value=relayCharacteristicPhase
  "Lookup table " : Subsystem
  MATLAB Function : MATLAB Function  TreatAsAtomicUnit=on
  Switch : Switch  Threshold=7  SaturateOnIntegerOverflow=off  InputSameDT=off
  Operating Time : Outport
  wires:
  Switch/1 -> Operating Time/1
  plugSetting/1 -> MATLAB Function/1(plugSetting)
  Constant9/1 -> Switch/2
  Constant/1 -> MATLAB Function/2(timeSetting)
  Constant3/1 -> MATLAB Function/3(relayCharacteristic)
  MATLAB Function/1(operatingTime) -> Switch/3
  "Lookup table "/1(Operating Time) -> Switch/1
  Current/1 -> "Lookup table "/1(Current)

== system RemoteMicrogrid/Operator Control Room/Microgrid Control/Protection & Power Tracking/Overcurrent relay/Earth Protection Unit/Operating Time/Lookup table ==
  Current : Inport
  2-D Lookup Table1 : Lookup_n-D  BreakpointsForDimension1=currentEarth  BreakpointsForDimension2=tmsEarth  Table=topEarth  InterpMethod=Cubic spline  ExtrapMethod=Cubic spline  InternalRulePriority=Speed  RndMeth=Simplest
      settings: InputPortMap=u0,u1
  Constant13 : Constant  Value=ethTimeSetting
  Constant16 : Constant  Value=topEarthActual
  Constant17 : Constant  Value=relayCharacteristicEarth
  Switch4 : Switch  Threshold=8  SaturateOnIntegerOverflow=off  InputSameDT=off
  Oeprating Time : Outport
  wires:
  Current/1 -> 2-D Lookup Table1/1
  Constant17/1 -> Switch4/2
  2-D Lookup Table1/1 -> Switch4/1
  Constant16/1 -> Switch4/3
  Constant13/1 -> 2-D Lookup Table1/2
  Switch4/1 -> Oeprating Time/1

== system RemoteMicrogrid/Operator Control Room/Microgrid Control/Protection & Power Tracking/Overcurrent relay/Phase Protection Unit/Operating time /Lookup table  ==
  Current : Inport
  2-D Lookup Table : Lookup_n-D  BreakpointsForDimension1=currentPhase  BreakpointsForDimension2=tmsPhase  Table=topPhase  InterpMethod=Cubic spline  ExtrapMethod=Cubic spline  InternalRulePriority=Speed  RndMeth=Simplest
      settings: InputPortMap=u0,u1
  Constant12 : Constant  Value=phTimeSetting  VectorParams1D=off
  Constant14 : Constant  Value=topPhaseActual
  Constant15 : Constant  Value=relayCharacteristicPhase
  Demux2 : Demux  Outputs=3
  Max : MinMax  Function=max  Inputs=3
  Switch3 : Switch  Threshold=8  SaturateOnIntegerOverflow=off  InputSameDT=off
  Operating Time : Outport
  wires:
  Constant15/1 -> Switch3/2
  Current/1 -> Demux2/1
  Constant12/1 -> 2-D Lookup Table/2
  Demux2/2 -> Max/2
  Demux2/1 -> Max/1
  Constant14/1 -> Switch3/3
  2-D Lookup Table/1 -> Switch3/1
  Demux2/3 -> Max/3
  Switch3/1 -> Operating Time/1
  Max/1 -> 2-D Lookup Table/1

== stateflow chart RemoteMicrogrid/Diesel Substation, BESS, & Microgrid Controller/Microgrid Controller/Microgrid Supervisory Control/Transition and Dispatch Control/On.Planned_Islanding ==
  state Enable
    plannedIslanding = true;
  state BreakerOpen
    PCC = 1;
    plannedIslandingStatus = true;
    plannedIslandingDispatch = true;
  (default) -> Enable
  Enable -> BreakerOpen : after(PlannedIslanding.delay,sec)[PlannedIslanding.status == true]
  data: PlannedIslanding input Bus: PlannedIslanding; PCC output; plannedIslanding output boolean; plannedIslandingDispatch output boolean; plannedIslandingStatus output boolean

== stateflow chart RemoteMicrogrid/Diesel Substation, BESS, & Microgrid Controller/Microgrid Controller/Microgrid Supervisory Control/Transition and Dispatch Control ==
  state On
    entry:
    Status.loadDispatch = false;
    Status.loadReference = 0;
    BrKControl.PCC = BreakerStatus;
    resyncDispatch = false;
    plannedIslandingDispatch = false;
    emergencyDispatch = false;
    state Steady_State_Grid_Connected
    state Steady_State_Islanded
    state Resynchronization
    state Unplanned_Islanding
    state Planned_Islanding
    (default) -> (junction 282)
    Steady_State_Grid_Connected -> (junction 317) : [PlannedIslanding.enable == true &&...
        |  BreakerStatus <=0]
    (junction 282) -> Steady_State_Grid_Connected [order 2] : [BreakerStatus <= 0 && ...
        | PlannedIslanding.enable == false]
    (junction 317) -> (junction 338)
    (junction 282) -> Steady_State_Islanded [order 1] : [BreakerStatus > 0 && ...
        | Resync.enable == false]
    (junction 282) -> (junction 312) [order 3]
    Steady_State_Islanded -> (junction 314) : [Resync.enable == true && ...
        | BreakerStatus > 0]
    (junction 314) -> (junction 329)
    Resynchronization -> Steady_State_Grid_Connected : [BreakerStatus <= 0 && ...
        | (Island.voltage > lowerVoltageLimit && ...
        | Island.voltage < upperVoltageLimit) && ...
        | (Island.frequency > lowerFrequencyLimit  && ...
        | Island.frequency  <  upperFrequencyLimit)]
    (junction 299) -> Steady_State_Islanded
    (junction 306) -> (junction 299)
    (junction 326) -> Resynchronization
    (junction 330) -> (junction 326)
    Unplanned_Islanding -> (junction 306) : [BreakerStatus > 0 && ...
        | (Island.voltage > lowerVoltageLimit && ...
        | Island.voltage < upperVoltageLimit) && ...
        | (Island.frequency > lowerFrequencyLimit  && ...
        | Island.frequency  <  upperFrequencyLimit)]
    (junction 312) -> Unplanned_Islanding [order 3]
    (junction 312) -> Resynchronization [order 1] : [Resync.enable == true && ...
        | BreakerStatus > 0]
    (junction 312) -> (junction 297) [order 2]
    (junction 285) -> (junction 306)
    On -> Unplanned_Islanding : [UnplannedIslandingEnable  > 0 && emergencyDispatch == false]
    (junction 297) -> Planned_Islanding : [PlannedIslanding.enable == true &&...
        | BreakerStatus <= 0 ]
    Planned_Islanding -> (junction 285) : [BreakerStatus > 0 && ...
        | (Island.voltage > lowerVoltageLimit && ...
        | Island.voltage < upperVoltageLimit) && ...
        | (Island.frequency > lowerFrequencyLimit  && ...
        | Island.frequency  <  upperFrequencyLimit)]
    (junction 341) -> Planned_Islanding
    (junction 329) -> (junction 330)
    (junction 338) -> (junction 341)
  (default) -> On
  data: LoadF2A function_output; resyncDispatch function_input; LoadF2B function_output; loadDispatch function_output; loadReference function_output; emergencyDispatch function_output; LoadF2A function_output; LoadF2B function_output; loadDispatch function_output; plannedIslandingDispatch function_input; emergencyDispatch function_output; PCC function_output; resync function_output; resyncDispatch function_output; resyncStatus function_output; PCC function_output; loadDispatch function_output; loadF2A function_output; loadF2B function_output; emergencyDispatch function_output; PCC function_output; plannedIslanding function_output; plannedIslandingDispatch function_output; plannedIslandingStatus function_output; Resync input Bus: Resync; UnplannedIslandingEnable input; Island input Bus: Island; lowerVoltageLimit parameter; upperFrequencyLimit parameter; upperVoltageLimit parameter; BrKControl output Bus: BrKControl; Status output Bus: Status; BreakerStatus input; PlannedIslanding input Bus: PlannedIslanding; lowerFrequencyLimit parameter; resyncDispatch local boolean size=1; plannedIslandingDispatch local boolean size=1; Transition_and_Dispatch_ControlMode output Enum: MicrogridStatus; emergencyDispatch local boolean size=1

== matlab function RemoteMicrogrid/Operator Control Room/Microgrid Control/Protection & Power Tracking/Overcurrent relay/Earth Protection Unit/Operating Time/Standard Characteristics ==
  data: plugSetting input; operatingTime output; timeSetting input; relayCharacteristic input
function operatingTime = fcn(plugSetting,timeSetting,relayCharacteristic)
   if plugSetting>1             % Fault condition
    switch relayCharacteristic  % Selection of relay characteristic
        case 1                  % IEC Normal Inverse
          a=0.14;      
          b=0.02;
          c=0;
        case 2                  % IEC Very Inverse
           a=13.5;
           b=1;
           c=0;
        case 3                  % IEC Extremely Inverse
            a=80;
            b=2;
            c=0;
        case 4                  % IEC Moderately Inverse
            a=0.0515;
            b=0.02;
            c=0.114;
        case 5                  % IEEE Very Inverse
            a=19.61;
            b=2;
            c=0.491;
        case 6                  % IEEE Exteremely Inverse
            a=28.2;
            b=2;
            c=0.1217;
        otherwise               % Definite Time
            a=1;
            b=1;
            c=0;
            plugSetting=2;
    end               
         operatingTime=timeSetting*(a/(power(max(plugSetting),b)-1)+c);  % Calculate the oeprating time of the relay    
   else
       operatingTime=inf;  % Set relay operating time to infinite if there is no fault
   end
end
